simulink model "ModuloHalfCell"  (R2018b)
settings: Solver=ode23tb  StartTime=0.0  StopTime=3  FixedStep=Ts_Power  RelTol=1e-4
PreLoadFcn:
  | Ts_Power=50e-6;
  | Slope_Vdc=1;
InitFcn:
  | Ts_Power=50e-6;
  | Tc=1e-5;%break algebraic loop time constant
  | BlockName=[gcs,'/PV cells 1-20'];
  | ModuleName=get_param(BlockName,'ModuleName');
  | Voc1=str2num(get_param(BlockName,'Voc'));
  | Nser1=str2num(get_param(BlockName,'Nser'));
  | Slope_Vdc=Nser1*Voc1;
StopFcn:
  | if exist('I','var') && exist('V','var')
  |    figure(1)
  |    clf
  |    n=find(I>=0);
  |    n=n(end);
  |    Vglobal=V(1:n);
  |    Iglobal=I(1:n);
  | 
  | 
  |    Pglobal=Vglobal.*Iglobal;
  |    n=find(Pglobal==max(Pglobal));
  |    Pmax=Pglobal(n);
  |    Vmp=Vglobal(n);
  |    Imp=Iglobal(n);
  | 
  | 
  |    subplot(211)
  |    plot(Vglobal, Iglobal,Vmp,Imp,'or')
  |    ylabel('Current (A)')
  |    title(sprintf('Global I-V & P-V characteristics\n %s' ,ModuleName))
  | 
  | 
  |    subplot(212)
  |    plot(Vglobal, Pglobal,Vmp,Pmax,'or')
  |    ylabel('Power (W)')
  |    xlabel('Voltage (V)')
  | end
libraries: powerlib x7, re_lib x6, simulink x1
Description:
  | Copyright 2008-2018 The MathWorks, Inc.
settings Model: Creator=MathWorks  LastModifiedBy=ricar
settings SolverCC: AlgebraicLoopSolver=LineSearch
settings DataIOCC: LimitDataPoints=on  SaveFormat=Array  SignalLoggingSaveFormat=ModelDataLogs
settings OptimizationCC: ExpressionDepthLimit=2147483647  LifeSpan=inf
settings DebuggingCC: UnderspecifiedInitializationDetection=Classic  MergeDetectMultiDrivingBlocksExec=none  SolverPrmCheckMsg=warning  FcnCallInpInsideContextMsg=warning  AllowSymbolicDim=off  StateNameClashWarn=warning  SFUnexpectedBacktrackingDiag=warning  SFNoUnconditionalDefaultTransitionDiag=warning  SFExecutionAtInitializationDiag=none
settings HardwareCC: ProdBitPerPointer=32  ProdBitPerSizeT=32  ProdBitPerPtrDiffT=32  ProdLargestAtomicFloat=None  ProdIntDivRoundTo=Undefined  ProdEndianess=Unspecified  ProdWordSize=32  ProdHWDeviceType=32-bit Generic
settings ModelReferenceCC: PropagateSignalLabelsOutOfModel=off
settings SFSimCC: SimUseLocalCustomCode=off
settings RTWCC: RTWUseLocalCustomCode=off
settings CodeAppCC: StateflowObjectComments=on
settings GRTTargetCC: TargetLangStandard=C89/C90 (ANSI)  GeneratePreprocessorConditionals=Disable all  CombineOutputUpdateFcns=off  GRTInterface=on
settings ConfigComp: CovMetricSettings=dw  CovHtmlReporting=on  CovSaveCumulativeToWorkspaceVar=on  CovSaveSingleToWorkspaceVar=on  CovExternalEMLEnable=off  CovSFcnEnable=off
settings SimscapeCC: SimscapeNormalizeSystem=off

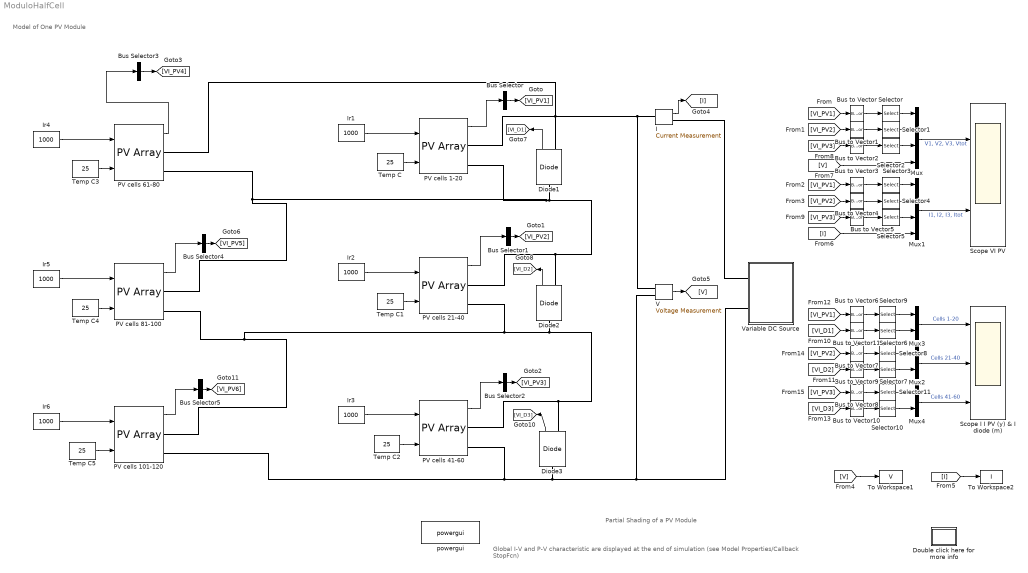
== system ModuloHalfCell ==
  note: Global I-V and P-V characteristic are displayed at the end of simulation
      | (see Model Properties/Callback StopFcn)
  note: Partial Shading of a PV Module
  note: Model of One PV Module
  Bus Selector{,1..5} (6 alike) : BusSelector  OutputSignals=V_PV,I_PV  OutputAsBus=on
  Bus to Vector{,1..11} (12 alike) : BusToVector
  Diode1 : powerlib/Power Electronics/Diode  Ron=0.001  Lon=0  Vf=0.7  IC=0  UseSnubber=off  Rs=1e5*inf  Cs=inf  Measurements=on
      settings: SourceProductName=Simscape Electrical
  Diode2 : powerlib/Power Electronics/Diode  Ron=0.001  Lon=0  Vf=0.7  IC=0  UseSnubber=off  Rs=1e5*inf  Cs=inf  Measurements=on
      settings: SourceProductName=Simscape Electrical
  Diode3 : powerlib/Power Electronics/Diode  Ron=0.001  Lon=0  Vf=0.7  IC=0  UseSnubber=off  Rs=1e5*inf  Cs=inf  Measurements=on
      settings: SourceProductName=Simscape Electrical
  Double click here for more info : Subsystem
      settings: OpenFcn=showdemo(bdroot(gcb))
      mask Display: disp('?')
  I : powerlib/Measurements/Current Measurement  PhasorSimulation=off  OutputType=Complex  PSBequivalent=0
      settings: SourceProductName=Simscape Electrical
  Ir{1..6} (6 alike) : Constant  Value=1000
  Mux : Mux
  Mux1 : Mux
  Mux2 : Mux  Inputs=2
  Mux3 : Mux  Inputs=2
  Mux4 : Mux  Inputs=2
  PV cells 1-20 : re_lib/Solar/PV Array  Npar=1  Nser=1  PlotType=array @ 25 deg.C & specified irradiances  S_vec="[ 1000  500  100 ]"  Temp_C_vec="[ 45 25  ]"  ModuleName=User-defined  PlotWhenSelected=off  Pm=74.9976  Ncell=20  Voc=41.18*20/60  Isc=13.85/2  Vm=33.91*20/60  Im=13.27/2  beta_Voc_pc=-0.28  alpha_Isc_pc=0.048  beta_Voc=-0.038435  alpha_Isc=0.003324  IL=6.9832  I0=1.008e-11  nI=0.98017  Rsh=199.2614  Rs=0.13145  BAL=on  Tc=Tc  Tfilter=5e-5
      settings: SourceProductName=Simscape Electrical
  PV cells 101-120 : re_lib/Solar/PV Array  Npar=1  Nser=1  PlotType=array @ 25 deg.C & specified irradiances  S_vec="[ 1000  500  100 ]"  Temp_C_vec="[ 45 25  ]"  ModuleName=User-defined  PlotWhenSelected=off  Pm=74.9976  Ncell=20  Voc=41.18*20/60  Isc=13.85/2  Vm=33.91*20/60  Im=13.27/2  beta_Voc_pc=-0.28  alpha_Isc_pc=0.048  beta_Voc=-0.038435  alpha_Isc=0.003324  IL=6.9832  I0=1.008e-11  nI=0.98017  Rsh=199.2614  Rs=0.13145  BAL=on  Tc=Tc  Tfilter=5e-5
      settings: SourceProductName=Simscape Electrical
  PV cells 21-40 : re_lib/Solar/PV Array  Npar=1  Nser=1  PlotType=array @ 25 deg.C & specified irradiances  S_vec="[ 1000  500  100 ]"  Temp_C_vec="[ 45 25  ]"  ModuleName=User-defined  PlotWhenSelected=off  Pm=74.9976  Ncell=20  Voc=41.18*20/60  Isc=13.85/2  Vm=33.91*20/60  Im=13.27/2  beta_Voc_pc=-0.28  alpha_Isc_pc=0.048  beta_Voc=-0.038435  alpha_Isc=0.003324  IL=6.9832  I0=1.008e-11  nI=0.98017  Rsh=199.2614  Rs=0.13145  BAL=on  Tc=Tc  Tfilter=5e-5
      settings: SourceProductName=Simscape Electrical
  PV cells 41-60 : re_lib/Solar/PV Array  Npar=1  Nser=1  PlotType=array @ 25 deg.C & specified irradiances  S_vec="[ 1000  500  100 ]"  Temp_C_vec="[ 45 25  ]"  ModuleName=User-defined  PlotWhenSelected=off  Pm=74.9976  Ncell=20  Voc=41.18*20/60  Isc=13.85/2  Vm=33.91*20/60  Im=13.27/2  beta_Voc_pc=-0.28  alpha_Isc_pc=0.048  beta_Voc=-0.038435  alpha_Isc=0.003324  IL=6.9832  I0=1.008e-11  nI=0.98017  Rsh=199.2614  Rs=0.13145  BAL=on  Tc=Tc  Tfilter=5e-5
      settings: SourceProductName=Simscape Electrical
  PV cells 61-80 : re_lib/Solar/PV Array  Npar=1  Nser=1  PlotType=array @ 25 deg.C & specified irradiances  S_vec="[ 1000  500  100 ]"  Temp_C_vec="[ 45 25  ]"  ModuleName=User-defined  PlotWhenSelected=off  Pm=74.9976  Ncell=20  Voc=41.18*20/60  Isc=13.85/2  Vm=33.91*20/60  Im=13.27/2  beta_Voc_pc=-0.28  alpha_Isc_pc=0.048  beta_Voc=-0.038435  alpha_Isc=0.003324  IL=6.9832  I0=1.008e-11  nI=0.98017  Rsh=199.2614  Rs=0.13145  BAL=on  Tc=Tc  Tfilter=5e-5
      settings: SourceProductName=Simscape Electrical
  PV cells 81-100 : re_lib/Solar/PV Array  Npar=1  Nser=1  PlotType=array @ 25 deg.C & specified irradiances  S_vec="[ 1000  500  100 ]"  Temp_C_vec="[ 45 25  ]"  ModuleName=User-defined  PlotWhenSelected=off  Pm=74.9976  Ncell=20  Voc=41.18*20/60  Isc=13.85/2  Vm=33.91*20/60  Im=13.27/2  beta_Voc_pc=-0.28  alpha_Isc_pc=0.048  beta_Voc=-0.038435  alpha_Isc=0.003324  IL=6.9832  I0=1.008e-11  nI=0.98017  Rsh=199.2614  Rs=0.13145  BAL=on  Tc=Tc  Tfilter=5e-5
      settings: SourceProductName=Simscape Electrical
  Scope I I PV (y) & I diode (m) : Scope  NumInputPorts=3
  Scope VI PV : Scope  NumInputPorts=2
  Selector{,1..2,6..7,10} (6 alike) : Selector  InputPortWidth=2  IndexOptions=Index vector (dialog)  Indices=[1]  OutputSizes=1
  Selector{3..5,8..9,11} (6 alike) : Selector  InputPortWidth=2  IndexOptions=Index vector (dialog)  Indices=[2]  OutputSizes=1
  Temp C{,1..5} (6 alike) : Constant  Value=25
  To Workspace1 : ToWorkspace  VariableName=V  SampleTime=1e-3
  To Workspace2 : ToWorkspace  VariableName=I  SampleTime=1e-3
  V : powerlib/Measurements/Voltage Measurement  PhasorSimulation=off  OutputType=Complex  PSBequivalent=0
      settings: SourceProductName=Simscape Electrical
  Variable DC Source : Subsystem
  powergui : powerlib/powergui  Priority=1  SimulationMode=Continuous  SampleTime=Ts_Power*0 + 20e-6  frequency=60  Iterations=50  frequencyindice=0  Pbase=100e6  ErrMax=1e-4  UnitsV=kV  UnitsW=MW  buscounter=0  FunctionMessages=off  echomessages=off  EnableUseOfTLC=off  CurrentSourceSwitches=on  DisableSnubberDevices=on  DisableRonSwitches=off  DisableVfSwitches=off  DisplayEquations=off  SolverType=Tustin/Backward Euler (TBE)  Interpol=off  ExternalGateDelay=off  methode=off  Ts=0  x0status=blocks  SPID=off  SwTol=0  HookPort=off  RestoreLinks=warning  ResistiveCurrentMeasurement=off  Frange=[0:2:500]  Ylog=off  Xlog=on  ShowGrid=off  save=off  variable=ZData  structure=0  ZoomFFT=on  StartTime=0.0  cycles=1  DisplayStyle=1  fundamental=60  FreqAxis=off  MaxFrequency=1000  frequencyindicesteady=1  RmsSteady=1  display=off
  wires:
  Ir1/1 -> PV cells 1-20/1
  Temp C/1 -> PV cells 1-20/2
  Ir2/1 -> PV cells 21-40/1
  Temp C1/1 -> PV cells 21-40/2
  I/1 -> [I]
  V/1 -> [V]
  Ir3/1 -> PV cells 41-60/1
  Temp C2/1 -> PV cells 41-60/2
  Diode1/1 -> [VI_D1]
  Diode2/1 -> [VI_D2]
  Diode3/1 -> [VI_D3]
  PV cells 1-20/1 -> Bus Selector/1
  Bus Selector/1 -> [VI_PV1]
  Bus Selector1/1 -> [VI_PV2]
  PV cells 21-40/1 -> Bus Selector1/1
  Bus Selector2/1 -> [VI_PV3]
  PV cells 41-60/1 -> Bus Selector2/1
  Mux/1 -> Scope VI PV/1  "V1, V2, V3, Vtot"
  [V] -> Mux/4
  [VI_PV1] -> Bus to Vector/1
  [VI_PV2] -> Bus to Vector1/1
  [VI_PV3] -> Bus to Vector2/1
  Selector/1 -> Mux/1
  Selector1/1 -> Mux/2
  Selector2/1 -> Mux/3
  Mux1/1 -> Scope VI PV/2  "I1, I2, I3, Itot"
  [I] -> Mux1/4
  [VI_PV1] -> Bus to Vector3/1
  [VI_PV2] -> Bus to Vector4/1
  [VI_PV3] -> Bus to Vector5/1
  Selector3/1 -> Mux1/1
  Selector4/1 -> Mux1/2
  Selector5/1 -> Mux1/3
  [VI_PV1] -> Bus to Vector6/1
  Mux3/1 -> Scope I I PV (y) & I diode (m)/1  "Cells 1-20"
  Selector9/1 -> Mux3/1
  [VI_D1] -> Bus to Vector11/1
  Selector6/1 -> Mux3/2
  [VI_PV2] -> Bus to Vector7/1
  Mux2/1 -> Scope I I PV (y) & I diode (m)/2  "Cells 21-40"
  Selector8/1 -> Mux2/1
  [VI_D2] -> Bus to Vector9/1
  Selector7/1 -> Mux2/2
  [VI_PV3] -> Bus to Vector8/1
  Mux4/1 -> Scope I I PV (y) & I diode (m)/3  "Cells 41-60"
  Selector11/1 -> Mux4/1
  [VI_D3] -> Bus to Vector10/1
  Selector10/1 -> Mux4/2
  [V] -> To Workspace1/1
  [I] -> To Workspace2/1
  Bus to Vector/1 -> Selector/1
  Bus to Vector1/1 -> Selector1/1
  Bus to Vector2/1 -> Selector2/1
  Bus to Vector3/1 -> Selector3/1
  Bus to Vector4/1 -> Selector4/1
  Bus to Vector5/1 -> Selector5/1
  Bus to Vector6/1 -> Selector9/1
  Bus to Vector7/1 -> Selector8/1
  Bus to Vector8/1 -> Selector11/1
  Bus to Vector9/1 -> Selector7/1
  Bus to Vector10/1 -> Selector10/1
  Bus to Vector11/1 -> Selector6/1
  Bus Selector5/1 -> [VI_PV6]
  PV cells 81-100/1 -> Bus Selector4/1
  Bus Selector4/1 -> [VI_PV5]
  Bus Selector3/1 -> [VI_PV4]
  Temp C5/1 -> PV cells 101-120/2
  PV cells 101-120/1 -> Bus Selector5/1
  Ir4/1 -> PV cells 61-80/1
  Temp C3/1 -> PV cells 61-80/2
  Ir5/1 -> PV cells 81-100/1
  Ir6/1 -> PV cells 101-120/1
  PV cells 61-80/1 -> Bus Selector3/1
  Temp C4/1 -> PV cells 81-100/2
  connections:
  PV cells 61-80/RConn1 -- PV cells 1-20/RConn1 -- Diode1/RConn1 -- V/LConn1 -- I/LConn1
  PV cells 21-40/RConn1 -- PV cells 61-80/RConn2 -- PV cells 81-100/RConn1 -- PV cells 1-20/RConn2 -- Diode1/LConn1 -- Diode2/RConn1
  I/RConn1 -- Variable DC Source/LConn1
  PV cells 81-100/RConn2 -- Diode2/LConn1 -- PV cells 41-60/RConn1 -- Diode3/RConn1 -- PV cells 21-40/RConn2 -- PV cells 101-120/RConn1
  PV cells 41-60/RConn2 -- Variable DC Source/LConn2 -- V/LConn2 -- Diode3/LConn1 -- PV cells 101-120/RConn2

== system ModuloHalfCell/Double click here for more info ==

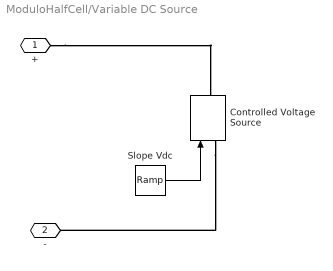
== system ModuloHalfCell/Variable DC Source ==
  Controlled Voltage Source : powerlib/Electrical Sources/Controlled Voltage Source  Initialize=on  Source_Type=AC  Amplitude=0  Phase=0  Frequency=0  Measurements=None
      settings: SourceProductName=Simscape Electrical
  Slope Vdc : simulink/Sources/Ramp  slope=Slope_Vdc  start=0  InitialOutput=0
  + : PMIOPort  Side=Left
  - : PMIOPort  Port=2  Side=Left
  wires:
  Slope Vdc/1 -> Controlled Voltage Source/1
  connections:
  Controlled Voltage Source/LConn1 -- -/RConn1
  +/RConn1 -- Controlled Voltage Source/RConn1
